simulink model "Full_State_Feedback_Question_A"  (R2016a)
settings: Solver=ode45  StartTime=0.0  StopTime=10.0  RelTol=1e-3
values from neighbouring files (symbols this model uses):
  A = [0,1,0,0;20.9,0,0,0;0,0,0,1;-0.8,0,0,0]    [SSAE_script.m]
  B = [0;-1;0;0.5]    [SSAE_script.m]
  C = [1,0,0,0;0,0,1,0]    [SSAE_script.m]
  K = place(A,B,poles)    [SSAE_script.m]
settings Model: Creator=el12074  LastModifiedBy=dimst
settings DataIOCC: LimitDataPoints=on  SaveFormat=Array
settings DebuggingCC: SolverPrmCheckMsg=warning
settings HardwareCC: ProdBitPerPointer=32  ProdLargestAtomicFloat=None  ProdIntDivRoundTo=Undefined  ProdEndianess=Unspecified  ProdWordSize=32  ProdHWDeviceType=32-bit Generic
settings ModelReferenceCC: PropagateSignalLabelsOutOfModel=off
settings ConfigComp: CovModelRefEnable=Off  CovSFcnEnable=off

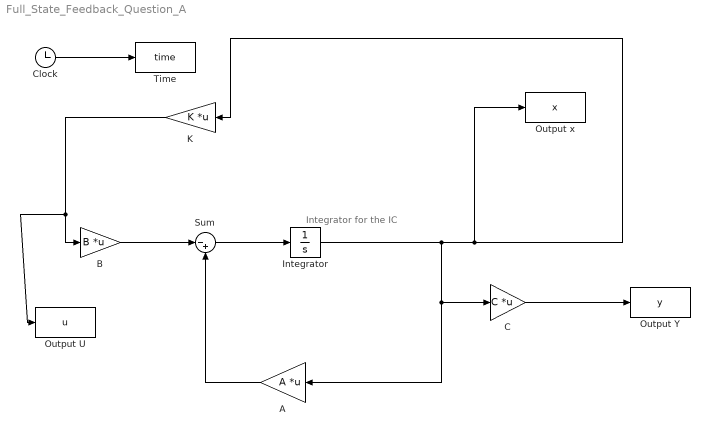
== system Full_State_Feedback_Question_A ==
  note: Integrator for the IC
  A : Gain  Gain=A  Multiplication=Matrix(K*u)
  B : Gain  Gain=B  Multiplication=Matrix(K*u)
  C : Gain  Gain=C  Multiplication=Matrix(K*u)
  Clock : Clock
  Integrator : Integrator  InitialCondition=[-0.2;-0.06;0.01;0.3]
  Output U : ToWorkspace  VariableName=u  SampleTime=-1
      settings: Save2DSignal=2-D array (concatenate along first dimension)
  Output Y : ToWorkspace  VariableName=y  SampleTime=-1
      settings: Save2DSignal=2-D array (concatenate along first dimension)
  Output x : ToWorkspace  VariableName=x  SampleTime=-1
      settings: Save2DSignal=2-D array (concatenate along first dimension)
  Sum : Sum  Inputs=|-+
  Time : ToWorkspace  VariableName=time  SampleTime=-1
      settings: Save2DSignal=2-D array (concatenate along first dimension)
  Κ : Gain  Gain=K  Multiplication=Matrix(K*u)
  wires:
  B/1 -> Sum/1
  A/1 -> Sum/2
  Sum/1 -> Integrator/1
  C/1 -> Output Y/1
  Clock/1 -> Time/1
  Integrator/1 -> Output x/1, Κ/1, A/1, C/1
  Κ/1 -> Output U/1, B/1
